simulink model "Sum14"  (Simulink 9.0)
settings: Solver=FixedStepAuto  StartTime=0.0  StopTime=10.0  FixedStep=0.1  RelTol=1e-3  EnableMultiTasking=on
settings Model: SuppressorTable=22 serialization::archive 11 0 6 0 0 0 0 0  Creator=arnaud  LastModifiedBy=hbourbou
settings DataIOCC: LimitDataPoints=on  SaveFormat=Structure  SignalLoggingSaveFormat=ModelDataLogs
settings OptimizationCC: ExpressionDepthLimit=2147483647
settings DebuggingCC: SolverPrmCheckMsg=warning  FcnCallInpInsideContextMsg=warning  StateNameClashWarn=warning  StrictBusMsg=Warning
settings GRTTargetCC: CombineOutputUpdateFcns=off  GRTInterface=on

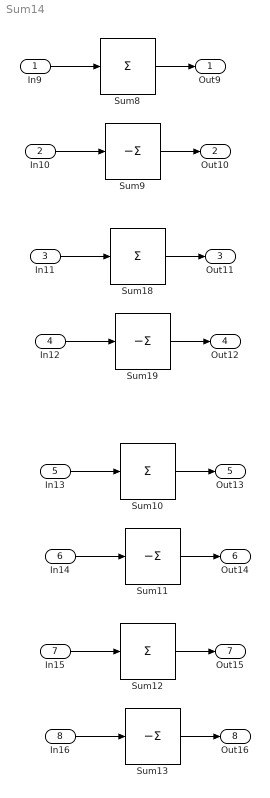
== system Sum14 ==
  In9 : Inport  OutDataTypeStr=int32
  In10 : Inport  Port=2  OutDataTypeStr=int32
  In11 : Inport  Port=3  OutDataTypeStr=int32  PortDimensions=3
  In12 : Inport  Port=4  OutDataTypeStr=int32  PortDimensions=3
  In13 : Inport  Port=5  OutDataTypeStr=int32  PortDimensions=[2 3]
  In14 : Inport  Port=6  OutDataTypeStr=int32  PortDimensions=[2 3]
  In15 : Inport  Port=7  OutDataTypeStr=int32  PortDimensions=[2 3]
  In16 : Inport  Port=8  OutDataTypeStr=int32  PortDimensions=[2 3]
  Sum10 : Sum  Inputs=+  CollapseMode=Specified dimension
  Sum11 : Sum  Inputs=-  CollapseMode=Specified dimension
  Sum12 : Sum  Inputs=+  CollapseMode=Specified dimension  CollapseDim=2
  Sum13 : Sum  Inputs=-  CollapseMode=Specified dimension  CollapseDim=2
  Sum18 : Sum  Inputs=+  CollapseMode=Specified dimension
  Sum19 : Sum  Inputs=-  CollapseMode=Specified dimension
  Sum8 : Sum  Inputs=+  CollapseMode=Specified dimension
  Sum9 : Sum  Inputs=-  CollapseMode=Specified dimension
  Out9 : Outport
  Out10 : Outport  Port=2
  Out11 : Outport  Port=3
  Out12 : Outport  Port=4
  Out13 : Outport  Port=5
  Out14 : Outport  Port=6
  Out15 : Outport  Port=7
  Out16 : Outport  Port=8
  wires:
  In9/1 -> Sum8/1
  Sum8/1 -> Out9/1
  In10/1 -> Sum9/1
  Sum9/1 -> Out10/1
  In11/1 -> Sum18/1
  Sum18/1 -> Out11/1
  In12/1 -> Sum19/1
  Sum19/1 -> Out12/1
  In13/1 -> Sum10/1
  Sum10/1 -> Out13/1
  In14/1 -> Sum11/1
  Sum11/1 -> Out14/1
  In15/1 -> Sum12/1
  Sum12/1 -> Out15/1
  In16/1 -> Sum13/1
  Sum13/1 -> Out16/1
